simulink model "joints"  (R2024a)
settings: Solver=VariableStepAuto  StartTime=0.0  StopTime=t  RelTol=1e-6  AbsTol=1e-9
values from neighbouring files (symbols this model uses):
  dtheta_0 = zeros(3, 1)    [main.m]
  g = [0 0 -9.80665]'    [main.m]
  K = [zeros(3, 3) zeros(3, 3) ... (first row only)    [main.m]
  L = [0.755 0.1269 0.083 0.083]'    [main.m]
  m = [7.538; 4.211; 1.202]    [main.m]
  m_p = 20    [main.m]
  theta_0 = zeros(3, 1)    [main.m]
settings Model: Creator=dzent  LastModifiedBy=dzent
settings DataIOCC: ExternalInput=[theta_d]'  SaveOutput=off  SignalLogging=off  DSMLogging=off  SaveTime=off  ReturnWorkspaceOutputs=off

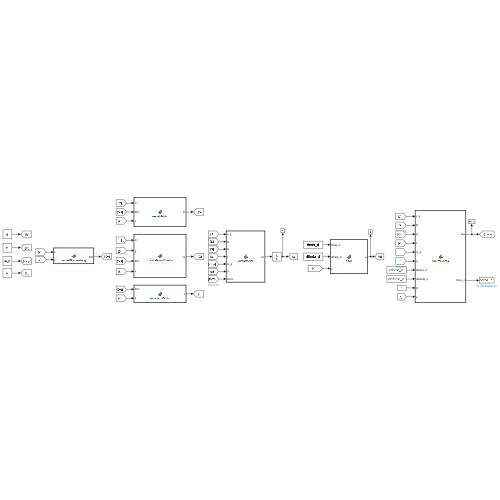
[thumbnail: Simulink's stored preview of the top-level diagram]
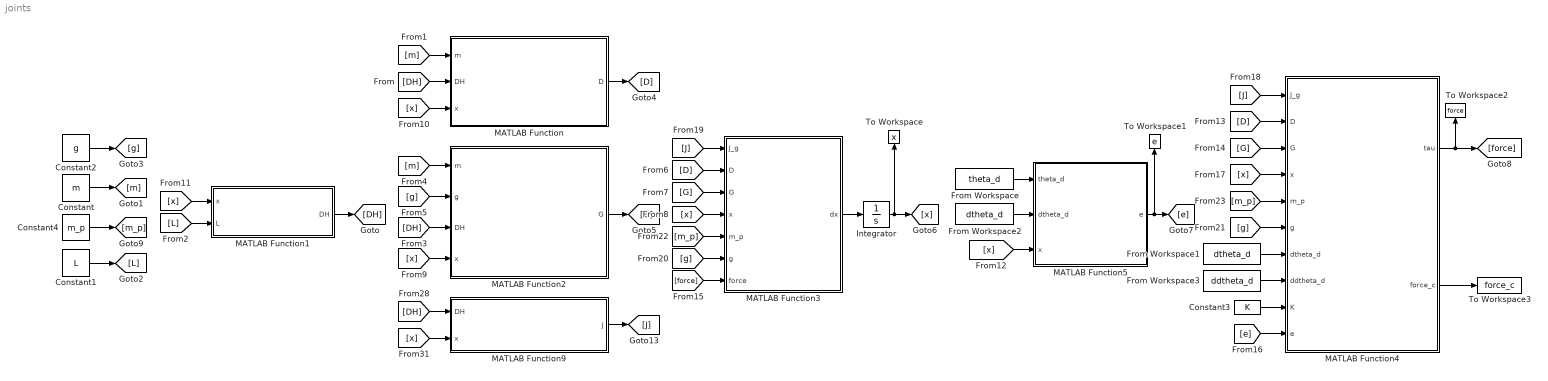
== system joints ==
  Constant : Constant  Value=m
  Constant1 : Constant  Value=L
  Constant2 : Constant  Value=g
  Constant3 : Constant  Value=K
  Constant4 : Constant  Value=m_p
  From Workspace : FromWorkspace  VariableName=theta_d
  From Workspace1 : FromWorkspace  VariableName=dtheta_d
  From Workspace2 : FromWorkspace  VariableName=dtheta_d
  From Workspace3 : FromWorkspace  VariableName=ddtheta_d
  Integrator : Integrator  InitialCondition=[theta_0; dtheta_0]  UpperSaturationLimit=[L(2 : end); inf; inf; inf]  LowerSaturationLimit=[zeros(3, 1); -inf; -inf; -inf]
  MATLAB Function : MATLAB Function  TreatAsAtomicUnit=on
  MATLAB Function1 : MATLAB Function  TreatAsAtomicUnit=on
  MATLAB Function2 : MATLAB Function  TreatAsAtomicUnit=on
  MATLAB Function3 : MATLAB Function  TreatAsAtomicUnit=on
  MATLAB Function4 : MATLAB Function  TreatAsAtomicUnit=on
  MATLAB Function5 : MATLAB Function  TreatAsAtomicUnit=on
  MATLAB Function9 : MATLAB Function  TreatAsAtomicUnit=on
  To Workspace : ToWorkspace  VariableName=x  SaveFormat=Timeseries  SampleTime=-1
  To Workspace1 : ToWorkspace  VariableName=e  SaveFormat=Timeseries  SampleTime=-1
  To Workspace2 : ToWorkspace  VariableName=force  SaveFormat=Timeseries  SampleTime=-1
  To Workspace3 : ToWorkspace  VariableName=force_c  SaveFormat=Timeseries  SampleTime=-1
  wires:
  MATLAB Function1/1(DH) -> [DH]
  [DH] -> MATLAB Function/2(DH)
  Constant/1 -> [m]
  Constant1/1 -> [L]
  [m] -> MATLAB Function/1(m)
  [L] -> MATLAB Function1/2(L)
  [m] -> MATLAB Function2/1(m)
  [DH] -> MATLAB Function2/3(DH)
  Constant2/1 -> [g]
  [g] -> MATLAB Function2/2(g)
  MATLAB Function/1(D) -> [D]
  MATLAB Function2/1(G) -> [G]
  [D] -> MATLAB Function3/2(D)
  [G] -> MATLAB Function3/3(G)
  MATLAB Function3/1(dx) -> Integrator/1
  Integrator/1 -> To Workspace/1, [x]
  [x] -> MATLAB Function3/4(x)
  [force] -> MATLAB Function3/7(force)
  [x] -> MATLAB Function2/4(x)
  [x] -> MATLAB Function/3(x)
  [x] -> MATLAB Function1/1(x)
  [x] -> MATLAB Function5/3(x)
  MATLAB Function5/1(e) -> To Workspace1/1, [e]
  [D] -> MATLAB Function4/2(D)
  [G] -> MATLAB Function4/3(G)
  MATLAB Function4/1(tau) -> To Workspace2/1, [force]
  [e] -> MATLAB Function4/10(e)
  [x] -> MATLAB Function4/4(x)
  Constant3/1 -> MATLAB Function4/9(K)
  From Workspace/1 -> MATLAB Function5/1(theta_d)
  [J] -> MATLAB Function4/1(J_g)
  [x] -> MATLAB Function9/2(x)
  MATLAB Function9/1(J) -> [J]
  [DH] -> MATLAB Function9/1(DH)
  MATLAB Function4/2(force_c) -> To Workspace3/1
  From Workspace2/1 -> MATLAB Function5/2(dtheta_d)
  From Workspace1/1 -> MATLAB Function4/7(dtheta_d)
  From Workspace3/1 -> MATLAB Function4/8(ddtheta_d)
  [J] -> MATLAB Function3/1(J_g)
  [g] -> MATLAB Function3/6(g)
  [g] -> MATLAB Function4/6(g)
  Constant4/1 -> [m_p]
  [m_p] -> MATLAB Function3/5(m_p)
  [m_p] -> MATLAB Function4/5(m_p)

== matlab function joints/MATLAB Function1 ==
  data: x input; DH output; L input
function DH = denavitHartenberg(x, L)

% Denavit - Hartenberg parameters' table
DH = denavitHartenberg(x(1 : 3, :), L);

== matlab function joints/MATLAB Function ==
  data: m input; D output; DH input; x input
function D = massMatrix(m, DH, x)

% Mass matrix
D = massMatrixHTM(m, DH, x(1 : 3, :));

== matlab function joints/MATLAB Function2 ==
  data: m input; g input; G output; DH input; x input
function G = gravitationalEffects(m, g, DH, x)

% Gravitational Effects
G = gravitationalEffectsHTM(m, g, DH, x(1 : 3, :));

== matlab function joints/MATLAB Function3 ==
  data: J_g input; D input; G input; x input; m_p input; g input; dx output; force input
function dx = jointsModel(J_g, D, G, x, m_p, g, force)

% Torques generated by the plates
tau_p = m_p * transpose(J_g) * g;

% State space matrix
A = [zeros(3, 3) eye(3)
     zeros(3, 3) zeros(3, 3)];

% Nonlinear terms
Phi = [zeros(3, 1); D \ (tau_p - G)];

% Input matrix
B = [zeros(3, 3) zeros(3, 3)
     zeros(3, 3) inv(D)];

% Input vector
u = [zeros(3, 1); force];

% State space equation
dx = (A * x) + Phi + (B * u);

== matlab function joints/MATLAB Function4 ==
  data: J_g input; D input; G input; x input; m_p input; g input; tau output; dtheta_d input; ddtheta_d input; K input; e input; force_c output
function [tau, force_c] = controlJoints(J_g, D, G, x, m_p, g, dtheta_d, ddtheta_d, K, e)

% Torques generated by the plates
tau_p = m_p * transpose(J_g) * g;

% State space matrix
A = [zeros(3, 3) eye(3)
     zeros(3, 3) zeros(3, 3)];

% Nonlinear terms
Phi = [zeros(3, 1); D \ (tau_p - G)];

% Input matrix
B = [zeros(3, 3) zeros(3, 3)
     zeros(3, 3) inv(D)];

% Input vector
u = pinv(B) * ([dtheta_d; ddtheta_d] + (K * e) - (A * x) - Phi);

% Control function
tau = u(4 : end, :);

% Total force at the end - effector
force_c = inv(J_g)' * tau;

== matlab function joints/MATLAB Function5 ==
  data: theta_d input; dtheta_d input; x input; e output
function e = error(theta_d, dtheta_d, x)

% Error function
e = [theta_d - x(1 : 3, :); dtheta_d - x(4 : 6, :)];

== matlab function joints/MATLAB Function9 ==
  data: DH input; x input; J output
function J = jacobianMatrix(DH, x)

% Gravitational Effects
J = jacobianMatrixHTM(DH, x(1 : 3, :), 5);
